simulink model "mhe_nmpc"  (R2012b)
settings: Solver=ode45  StartTime=0.0  StopTime=5  RelTol=1e-3
settings Model: Creator=John  LastModifiedBy=John

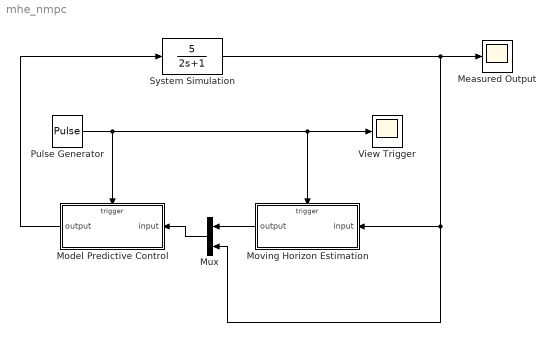
== system mhe_nmpc ==
  Measured Output : Scope
  Model Predictive Control : Subsystem  TreatAsAtomicUnit=on
  Moving Horizon Estimation : Subsystem  TreatAsAtomicUnit=on
  Mux : Mux  Inputs=2
  Pulse Generator : DiscretePulseGenerator  PulseType=Time based  Period=0.1  PulseWidth=10
  System Simulation : TransferFcn  Numerator=[5]  Denominator=[2 1]
  View Trigger : Scope
  wires:
  Pulse Generator/1 -> Model Predictive Control/Trigger, View Trigger/1, Moving Horizon Estimation/Trigger
  System Simulation/1 -> Moving Horizon Estimation/1(input), Mux/2, Measured Output/1
  Model Predictive Control/1(output) -> System Simulation/1
  Moving Horizon Estimation/1(output) -> Mux/1
  Mux/1 -> Model Predictive Control/1(input)

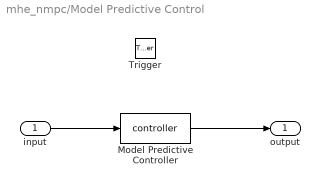
== system mhe_nmpc/Model Predictive Control ==
  input : Inport  PortDimensions=2
  Trigger : TriggerPort
  Model Predictive Controller : MATLABFcn  MATLABFcn=controller
  output : Outport  PortDimensions=1
  wires:
  input/1 -> Model Predictive Controller/1
  Model Predictive Controller/1 -> output/1

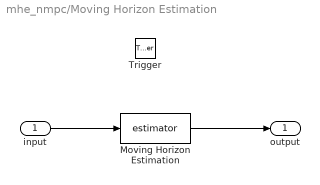
== system mhe_nmpc/Moving Horizon Estimation ==
  input : Inport  PortDimensions=1
  Trigger : TriggerPort
  Moving Horizon Estimation : MATLABFcn  MATLABFcn=estimator
  output : Outport  PortDimensions=1
  wires:
  input/1 -> Moving Horizon Estimation/1
  Moving Horizon Estimation/1 -> output/1
